simulink model "Charge_1_V1_experiment"  (R2018b)
settings: Solver=FixedStepDiscrete  StartTime=0.0  StopTime=1  FixedStep=0.001  RelTol=1e-3
PreLoadFcn:
  | librarySetup
  | eval([bdroot,'_startup']) %Calling [modelName]_startup.m
undefined symbols (not defined in the file or in its folder): A0, A1, Car1__Authorize, Car2_Authorize, CON2, CON3, CON4, Control_Mode_In, CurrentSP, D10, D12, D13, D2, D3, D4, D5, D6, D7, D8, Free_Charge, Frequency_High_Point, Frequency_Low_Point, Frequency_Mid_high, Frequency_Mid_low, HVol_High_Point, HVol_Low_Point, HVol_Mid_high, HVol_Mid_low, HVoltage_Factor, SeconCar_ThreePhase, V_Current_five, V_Current_four, V_Current_one, V_Current_six, V_Current_three, V_Current_two, V_Frequency, V_MaxPliot, V_MinPliot, Vol_High_Point, Vol_Low_Point, Vol_Mid_high, Vol_Mid_low, Voltage_Factor, Voltage_Mode_Test
libraries: simulink x324, HANcoder_STM32_Target x30, powerlib_meascontrol x8, simulink_extras x2
(part 1 of 13)
CloseFcn:
  | rtwprivate ssgencode ModelCloseRequest mytest
settings Model: Creator=Jason van Kolfschoten  LastModifiedBy=TrungNguyen
settings SolverCC: PositivePriorityOrder=on
settings DataIOCC: LimitDataPoints=on  SaveFormat=Array  SignalLoggingSaveFormat=ModelDataLogs  SaveOutput=off  SaveTime=off
settings OptimizationCC: BlockReduction=off  DefaultParameterBehavior=Inlined  InlineInvariantSignals=on  ExpressionDepthLimit=2147483647  StateBitsets=on  DataBitsets=on  ZeroExternalMemoryAtStartup=off  ZeroInternalMemoryAtStartup=off  InitFltsAndDblsToZero=on  NoFixptDivByZeroProtection=on  EfficientFloat2IntCast=on  LifeSpan=inf
settings DebuggingCC: SaveWithDisabledLinksMsg=none  SaveWithParameterizedLinksMsg=none  CheckSSInitialOutputMsg=off  UnderspecifiedInitializationDetection=Classic  MergeDetectMultiDrivingBlocksExec=none  SignalResolutionControl=TryResolveAll  SolverPrmCheckMsg=warning  InheritedTsInSrcMsg=none  MultiTaskDSMMsg=warning  MultiTaskCondExecSysMsg=none  ParameterPrecisionLossMsg=none  FcnCallInpInsideContextMsg=warning  StateNameClashWarn=warning  SFUnexpectedBacktrackingDiag=warning  SFNoUnconditionalDefaultTransitionDiag=warning  SFExecutionAtInitializationDiag=none
settings HardwareCC: ProdBitPerPointer=32  ProdBitPerSizeT=32  ProdBitPerPtrDiffT=32  ProdLargestAtomicFloat=None  ProdIntDivRoundTo=Undefined  ProdWordSize=32  ProdHWDeviceType=Generic->32-bit Embedded Processor  TargetEndianess=LittleEndian  TargetHWDeviceType=Infineon->TriCore
settings ModelReferenceCC: PropagateSignalLabelsOutOfModel=off
settings SFSimCC: SimUseLocalCustomCode=off  MATLABDynamicMemAlloc=off
settings RTWCC: SystemTargetFile=ert.tlc  MakeCommand=make_rtw SHELL= HANcoder_PORTABLE=1 HANcoder_BOOTLOADER=1  TemplateMakefile=STM32_E407_gcc.tmf  Description=Real-Time Workshop Embedded Coder (no auto configuration)  RTWUseLocalCustomCode=off
settings CodeAppCC: ForceParamTrailComments=on  IgnoreCustomStorageClasses=off  SimulinkDataObjDesc=on  CustomSymbolStrGlobalVar=rt$N$M  CustomSymbolStrType=$N$M  CustomSymbolStrFcn=$N$M$F  CustomSymbolStrMacro=$N$M  InsertBlockDesc=on  StateflowObjectComments=on  InternalIdentifier=Classic
settings ERTTargetCC: TargetFcnLib=ansi_tfl_tmw.mat  MultiwordLength=2048  IncludeMdlTerminateFcn=off  SuppressErrorStatus=on  SupportNonFinite=off  GenerateASAP2=on  InlinedParameterPlacement=NonHierarchical  ERTCustomFileTemplate=example_file_process.tlc  ConvertIfToSwitch=off  SuppressUnreachableDefaultCases=off  IndentSize=4
settings ConfigComp: CovMetricSettings=dw  CovHtmlReporting=on  CovSaveCumulativeToWorkspaceVar=on  CovSaveSingleToWorkspaceVar=on  CovExternalEMLEnable=off  DVMaxProcessTime=600  DVDisplayUnsatisfiableObjectives=on  DVAutomaticStubbing=off  DVModelCoverageObjectives=MCDC  DVMaxTestCaseSteps=500  DVTestSuiteOptimization=CombinedObjectives  DVDetectActiveLogic=on  DVSaveHarnessModel=on

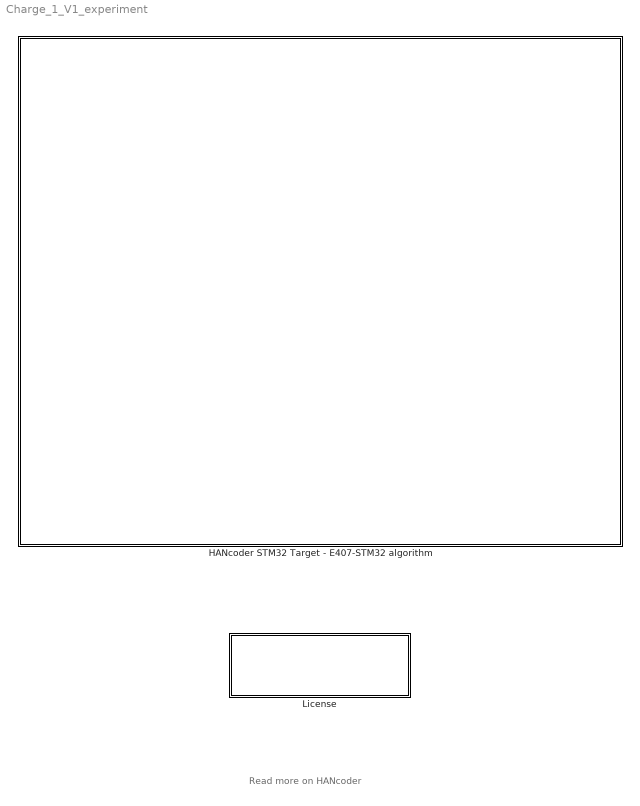
== system Charge_1_V1_experiment ==
  note: Read more on HANcoder
  HANcoder STM32 Target - E407-STM32 algorithm : Subsystem  mask(TopLevelSubsystem){}
      settings: CopyFcn=HANcoderChecks('Copy');  NameChangeFcn=HANcoderChecks('NameChangeE407');  MoveFcn=HANcoderChecks('MoveE407');
      mask Display: image(imread('STM32_E407_HAN.jpg'))
  License : Subsystem  mask(License){}
      settings: NameChangeFcn=HANcoderChecks('NameChangeLicenseBlock');  OpenFcn=winopen('License.pdf')  MoveFcn=HANcoderChecks('MoveLicenseBlock');
      mask Display: disp(['End-User License Agreement\n','please read before use']);

== system Charge_1_V1_experiment/HANcoder STM32 Target - E407-STM32 algorithm ==
  note: Chang current SP for each of charger
  note: Spare_Digital A4(from particle)
  Authorized card : Subsystem
  Car1 : Subsystem
  Car2 : Subsystem
  Config : Subsystem
  Counter Limited1 : simulink/Sources/Counter Limited  uplimit=20  tsamp=0.001
  Current_SP : Subsystem
  Delay : Delay  DelayLength=1  InitialCondition=0
  Delay1 : Delay  DelayLength=1  InitialCondition=0
  Energy Meter : Subsystem
  Partclie_SP_Receive : Subsystem
  Subsystem : Subsystem
  Terminator{,1..12} (13 alike) : Terminator
  wires:
  Current_SP/2(PWM_Out2) -> Car2/3(PWM_Signal)
  Delay1/1 -> Current_SP/18(Charge_state2)
  Car2/1(Out1) -> Delay1/1
  Current_SP/1(PWM_Out1) -> Car1/3(PWM_signal)
  Delay/1 -> Current_SP/17(Charge_state)
  Car1/1(state) -> Delay/1
  Counter Limited1/1 -> Partclie_SP_Receive/1(In1)
  Subsystem/2(V_Auth) -> Terminator2/1
  Subsystem/5(V_Current1) -> Terminator4/1
  Subsystem/6(V_Current2) -> Terminator5/1
  Subsystem/7(V_Current3) -> Terminator6/1
  Subsystem/8(V_Current4) -> Terminator7/1
  Subsystem/9(V_Current5) -> Terminator8/1
  Subsystem/10(V_Current6) -> Terminator9/1
  Subsystem/11(V_MaxPilot) -> Terminator10/1
  Subsystem/12(V_MinPilot) -> Terminator11/1
  Subsystem/4(2ndcarThreephase) -> Terminator3/1
  Authorized card/1(Sysstartcar1) -> Car1/1(System_Start)
  Authorized card/2(Sysstartcar2) -> Car2/1(" System_Start")
  Subsystem/3(V_Auth1) -> Terminator12/1
  Authorized card/3(RFID_Read) -> Car2/2(Read_RFID), Car1/2(RFID)
  Authorized card/4(2_Car_Connected) -> Current_SP/1(2_carConnected)
  Energy Meter/1(Current Phase 1) -> Current_SP/2(Cuurent1)
  Energy Meter/2(Current phase 2) -> Current_SP/3(Current2)
  Energy Meter/3(Current phase 3) -> Current_SP/4(Current3)
  Energy Meter/4(Current phase 4) -> Current_SP/5(Cuurent4)
  Energy Meter/5(Current phase 5) -> Current_SP/6(Current5)
  Energy Meter/6(Current phase 6) -> Current_SP/7(Current6)
  Energy Meter/7(vol1) -> Current_SP/8(vol1)
  Energy Meter/8(vol2) -> Current_SP/9(vol2)
  Energy Meter/9(vol3) -> Current_SP/10(vol3)
  Energy Meter/10(vol4) -> Current_SP/11(vol4)
  Energy Meter/11(vol5) -> Current_SP/12(vol5)
  Energy Meter/12(vol6) -> Current_SP/13(vol6)
  Partclie_SP_Receive/1(Particle_SP1) -> Current_SP/15(ParticleSP)
  Partclie_SP_Receive/2(Particle_SP2) -> Current_SP/16(ParticleSP2)
  Energy Meter/13(Fre) -> Terminator/1
  Subsystem/1(V_Fre) -> Current_SP/14(Frequency), Terminator1/1

== system Charge_1_V1_experiment/License ==

== system Charge_1_V1_experiment/HANcoder STM32 Target - E407-STM32 algorithm/Authorized card ==
  Constant : Constant  Value=Free_Charge  OutDataTypeStr=boolean  SampleTime=-1
  Digital Input : HANcoder_STM32_Target/STM32-E407/Digital Inputs/Digital Input  Tag=HANcoder_TARGET_STM32_E407  pinID=CON2 - A2 - 5V Tolerant  config=Floating  tsamp=0.01
      settings: SourceProductName=HANcoder STM32 Target
  Digital Input1 : HANcoder_STM32_Target/STM32-E407/Digital Inputs/Digital Input  Tag=HANcoder_TARGET_STM32_E407  pinID=CON2 - A3 - 5V Tolerant  config=Floating  tsamp=0.01
      settings: SourceProductName=HANcoder STM32 Target
  Digital Input2 : HANcoder_STM32_Target/STM32-E407/Digital Inputs/Digital Input  Tag=HANcoder_TARGET_STM32_E407  pinID=CON2 - A4 - 5V Tolerant  config=Floating  tsamp=0.001
      settings: SourceProductName=HANcoder STM32 Target
  Logical Operator : Logic  AllPortsSameDT=off  OutDataTypeStr=boolean
  Logical Operator1 : Logic  Operator=OR  AllPortsSameDT=off  OutDataTypeStr=boolean
  Logical Operator2 : Logic  Operator=OR  AllPortsSameDT=off  OutDataTypeStr=boolean
  Sysstartcar1 : Outport
  Sysstartcar2 : Outport  Port=2
  RFID_Read : Outport  Port=3
  2_Car_Connected : Outport  Port=4
  wires:
  Logical Operator2/1 -> Sysstartcar2/1, Logical Operator/1  "Enable_card2"
  Logical Operator1/1 -> Logical Operator/2, Sysstartcar1/1  "Enable_card1"
  Logical Operator/1 -> 2_Car_Connected/1
  Digital Input2/1 -> RFID_Read/1  "RFID_Read"
  Constant/1 -> Logical Operator2/1, Logical Operator1/2
  Digital Input/1 -> Logical Operator1/1
  Digital Input1/1 -> Logical Operator2/2

== system Charge_1_V1_experiment/HANcoder STM32 Target - E407-STM32 algorithm/Car1 ==
  note: Force system start and remove locking actuator
  System_Start : Inport
  RFID : Inport  Port=2
  PWM_signal : Inport  Port=3
  Chart1 : Stateflow chart  TreatAsAtomicUnit=on
  Motorlock controll : Subsystem
  Output leds : Subsystem
  PWM : Subsystem
  Pilotcar1 : Subsystem
  Terminator : Terminator
  Terminator1 : Terminator
  delaytime : Subsystem
  state : Outport
  wires:
  Chart1/2(Pwm) -> PWM/2(Current_SP)
  Pilotcar1/2(Charger_level_min) -> Chart1/2(Minvalue)
  PWM_signal/1 -> Chart1/3(inPWM)
  Pilotcar1/1(Charger_level_max) -> Chart1/1(Maxvalue)
  Chart1/1(Switch) -> Terminator/1, delaytime/1(In1)  "LockCar1On"
  System_Start/1 -> Chart1/4(Start)
  delaytime/1(Lockoutput) -> Terminator1/1  "LockCar1off"
  delaytime/2(Switch_output) -> PWM/1(Switch)  "SwitchCar1"
  Chart1/3(State) -> Output leds/1(State), state/1  "Car1State"
  RFID/1 -> Output leds/2(RFID)

== system Charge_1_V1_experiment/HANcoder STM32 Target - E407-STM32 algorithm/Car2 ==
  " System_Start" : Inport
  Read_RFID : Inport  Port=2
  PWM_Signal : Inport  Port=3
  Chart1 : Stateflow chart  TreatAsAtomicUnit=on
  Motorlock controll : Subsystem
  Output leds : Subsystem
  PWM : Subsystem
  Pilotcar2 : Subsystem
  Terminator : Terminator
  Terminator1 : Terminator
  delaytime : Subsystem
  Out1 : Outport
  wires:
  delaytime/2(Switch_output) -> PWM/1(Switch)  "SwitchCar2"
  delaytime/1(Lockoutput) -> Terminator1/1  "LockCar2off"
  " System_Start"/1 -> Chart1/4(Start)
  Chart1/1(Switch) -> Terminator/1, delaytime/1(In1)  "LockCar2On"
  Pilotcar2/1(Charger_level_max) -> Chart1/1(Maxvalue)  "Maxpilotcar2"
  PWM_Signal/1 -> Chart1/3(inPWM)
  Pilotcar2/2(Charger_level_min) -> Chart1/2(Minvalue)  "Minpilotcar2"
  Chart1/2(Pwm) -> PWM/2(Current_SP)
  Chart1/3(State) -> Out1/1, Output leds/1(State)  "Car2State"
  Read_RFID/1 -> Output leds/2(RFID)

== system Charge_1_V1_experiment/HANcoder STM32 Target - E407-STM32 algorithm/Config ==
  Base Sample Time config : HANcoder_STM32_Target/STM32-E407/System Config/Base Sample Time config  Tag=HANcoder_TARGET_STM32_E407  Description=HANcoder Target STM32-E407 blockset version 0.5  baseSampleTime=1  extraStack=5000
      settings: SourceProductName=HANcoder STM32 Target
  Build settings : HANcoder_STM32_Target/STM32-E407/System Config/Build settings  Tag=HANcoder_TARGET_STM32_E407  AutoASAP2add=on  AutoFlash=Ethernet
      settings: SourceProductName=HANcoder STM32 Target
  Custom ID config : HANcoder_STM32_Target/STM32-E407/System Config/Custom ID config  Tag=HANcoder_TARGET_STM32_E407  softID=softwareID  softNUM=1
      settings: SourceProductName=HANcoder STM32 Target
  Ethernet config : HANcoder_STM32_Target/STM32-E407/System Config/Ethernet config  Tag=HANcoder_TARGET_STM32_E407  ip1=169  ip2=254  ip3=19  ip4=63  nm1=255  nm2=255  nm3=0  nm4=0  gw1=169  gw2=254  gw3=1  gw4=1
      settings: SourceProductName=HANcoder STM32 Target
  System information : Subsystem
  XCP on TCP/IP config : HANcoder_STM32_Target/STM32-E407/System Config/XCP on TCP//IP config  Tag=HANcoder_TARGET_STM32_E407  port=1000
      settings: SourceProductName=HANcoder STM32 Target

== system Charge_1_V1_experiment/HANcoder STM32 Target - E407-STM32 algorithm/Current_SP ==
  note: When 2 car had been connected, current need to reduce to 16A first
  note: Control Mode: 1 : Particle SP
      | 			   2: Frequency
      | 			  3: Hantune_SP
      | 			  4: Free_Charge
      | 			  5: Voltage_Mode
  2_carConnected : Inport
  Cuurent1 : Inport  Port=2
  Current2 : Inport  Port=3
  Current3 : Inport  Port=4
  Cuurent4 : Inport  Port=5
  Current5 : Inport  Port=6
  Current6 : Inport  Port=7
  vol1 : Inport  Port=8
  vol2 : Inport  Port=9
  vol3 : Inport  Port=10
  vol4 : Inport  Port=11
  vol5 : Inport  Port=12
  vol6 : Inport  Port=13
  Frequency : Inport  Port=14
  ParticleSP : Inport  Port=15  OutDataTypeStr=single
  ParticleSP2 : Inport  Port=16  OutDataTypeStr=single
  Charge_state : Inport  Port=17
  Charge_state2 : Inport  Port=18
  Constant1 : Constant  Value=Control_Mode_In  OutDataTypeStr=single  SampleTime=0.01
  Current_Limit1 : Subsystem
  Subsystem1 : Subsystem
  Subsystem2 : Subsystem
  Voltage_input : Subsystem
  Voltage_input1 : Subsystem
  Voltage_testblock : Subsystem
  PWM_Out1 : Outport
  PWM_Out2 : Outport  Port=2
  wires:
  Subsystem1/1(PWM_Out1) -> PWM_Out1/1
  Charge_state/1 -> Subsystem1/9(Sys_charge)
  Charge_state2/1 -> Subsystem2/7(Sys_charge)
  Subsystem2/1(PWM_Out1) -> PWM_Out2/1
  Frequency/1 -> Subsystem2/8(Frequency)
  Constant1/1 -> Subsystem2/10(Control_Mode)  "Mode"
  2_carConnected/1 -> Current_Limit1/1(2_carConnected)
  Current_Limit1/4(Current_Limit) -> Subsystem2/1(Current_Limit)
  Cuurent1/1 -> Current_Limit1/2(In1)
  Current2/1 -> Current_Limit1/3(In2)
  Current3/1 -> Current_Limit1/4(In3)
  Current_Limit1/5(Frequency_Conditionnd) -> Subsystem2/2(Condition)
  ParticleSP2/1 -> Subsystem2/9(Particleinput)
  ParticleSP/1 -> Subsystem1/10(Particleenter1)
  Subsystem2/2(2carConnect_O) -> Subsystem1/4(2ndCarConnected)
  Subsystem2/3(Fre_O) -> Subsystem1/5(Frequency)
  Subsystem2/6(Control_Mode_Out) -> Subsystem1/8(Control_mode)
  Subsystem2/5(Condition_O) -> Subsystem1/7(Fre_Cond)
  Subsystem2/4(Current_Limit_O) -> Subsystem1/6(CurrenLimitCar1)
  Cuurent4/1 -> Current_Limit1/5(In4)
  Current5/1 -> Current_Limit1/6(In5)
  Current6/1 -> Current_Limit1/7(In6)
  Current_Limit1/6(Out4) -> Subsystem2/3(In4)
  Current_Limit1/7(Out5) -> Subsystem2/4(In5)
  Current_Limit1/8(Out6) -> Subsystem2/5(In6)
  Current_Limit1/9(2_carConnected_O) -> Subsystem2/6(2carConnect)
  Current_Limit1/1(Out1) -> Subsystem1/1(Phase1)
  Current_Limit1/2(Out2) -> Subsystem1/2(Phase2)
  Current_Limit1/3(Out3) -> Subsystem1/3(Phase3)
  Subsystem2/7(3phasecar2) -> Current_Limit1/9(3phasecar2)
  Subsystem1/2(3phasecar1) -> Current_Limit1/8(3phasecar1)
  vol2/1 -> Voltage_input/2(In2)
  vol3/1 -> Voltage_input/3(In3)
  vol4/1 -> ?
  vol5/1 -> Voltage_input1/2(In2)
  vol6/1 -> Voltage_input1/3(In3)
  Voltage_input/1(Out1) -> Subsystem1/11(Voltage)  "Voltage_level_check"
  Voltage_input1/1(Out1) -> Subsystem2/11(Voltage_in)  "Voltage_level_check_1"
  Voltage_testblock/1(Vol) -> Voltage_input1/1(In1), Voltage_input/1(In1)

== system Charge_1_V1_experiment/HANcoder STM32 Target - E407-STM32 algorithm/Energy Meter ==
  Counter Limited1 : simulink/Sources/Counter Limited  uplimit=1400  tsamp=0.001
  Energy_Meter : Subsystem
  Energy_Meter_Recieve : Subsystem
  Energymeter_Request : Subsystem
  Particle : Subsystem
  Current Phase 1 : Outport
  Current phase 2 : Outport  Port=2
  Current phase 3 : Outport  Port=3
  Current phase 4 : Outport  Port=4
  Current phase 5 : Outport  Port=5
  Current phase 6 : Outport  Port=6
  vol1 : Outport  Port=7
  vol2 : Outport  Port=8
  vol3 : Outport  Port=9
  vol4 : Outport  Port=10
  vol5 : Outport  Port=11
  vol6 : Outport  Port=12
  Fre : Outport  Port=13
  wires:
  Counter Limited1/1 -> Energy_Meter_Recieve/1(In1)
  Energy_Meter_Recieve/1(Current Phase 1) -> Current Phase 1/1
  Energy_Meter_Recieve/2(Current phase 2) -> Current phase 2/1
  Energy_Meter_Recieve/3(Current phase 3) -> Current phase 3/1
  Energy_Meter_Recieve/4(Current phase 4) -> Current phase 4/1
  Energy_Meter_Recieve/5(Current phase 5) -> Current phase 5/1
  Energy_Meter_Recieve/6(Current phase 6) -> Current phase 6/1
  Energy_Meter_Recieve/13(Frequency) -> Fre/1
  Energy_Meter_Recieve/7(vol1) -> vol1/1
  Energy_Meter_Recieve/8(vol2) -> vol2/1
  Energy_Meter_Recieve/12(vol6) -> vol6/1
  Energy_Meter_Recieve/11(vol5) -> vol5/1
  Energy_Meter_Recieve/10(vol4) -> vol4/1
  Energy_Meter_Recieve/9(vol3) -> vol3/1

== system Charge_1_V1_experiment/HANcoder STM32 Target - E407-STM32 algorithm/Partclie_SP_Receive ==
  In1 : Inport
  SP1 : Subsystem
  Particle_SP1 : Outport  OutDataTypeStr=single  SampleTime=0.1
  Particle_SP2 : Outport  Port=2  OutDataTypeStr=single  SampleTime=0.1
  wires:
  In1/1 -> SP1/1(In1)
  SP1/1(Out1) -> Particle_SP1/1
  SP1/2(Out2) -> Particle_SP2/1

== system Charge_1_V1_experiment/HANcoder STM32 Target - E407-STM32 algorithm/Subsystem ==
  Constant : Constant  Value=V_Frequency  OutDataTypeStr=single  SampleTime=-1
  Constant1 : Constant  Value=SeconCar_ThreePhase  SampleTime=-1
  Constant10 : Constant  Value=V_MinPliot  SampleTime=-1
  Constant11 : Constant  Value=Car2_Authorize  OutDataTypeStr=boolean  SampleTime=0.01
  Constant2 : Constant  Value=V_Current_one  SampleTime=-1
  Constant3 : Constant  Value=V_Current_two  SampleTime=-1
  Constant4 : Constant  Value=V_Current_three  SampleTime=-1
  Constant5 : Constant  Value=V_Current_four  SampleTime=-1
  Constant6 : Constant  Value=V_Current_five  SampleTime=-1
  Constant7 : Constant  Value=V_Current_six  SampleTime=-1
  Constant8 : Constant  Value=Car1__Authorize  OutDataTypeStr=boolean  SampleTime=0.01
  Constant9 : Constant  Value=V_MaxPliot  SampleTime=-1
  Fre_testblock : Subsystem
  Terminator : Terminator
  V_Fre : Outport
  V_Auth : Outport  Port=2
  V_Auth1 : Outport  Port=3
  2ndcarThreephase : Outport  Port=4
  V_Current1 : Outport  Port=5
  V_Current2 : Outport  Port=6
  V_Current3 : Outport  Port=7
  V_Current4 : Outport  Port=8
  V_Current5 : Outport  Port=9
  V_Current6 : Outport  Port=10
  V_MaxPilot : Outport  Port=11
  V_MinPilot : Outport  Port=12
  wires:
  Constant/1 -> Terminator/1
  Constant8/1 -> V_Auth/1
  Constant1/1 -> 2ndcarThreephase/1
  Constant2/1 -> V_Current1/1
  Constant3/1 -> V_Current2/1
  Constant4/1 -> V_Current3/1
  Constant5/1 -> V_Current4/1
  Constant6/1 -> V_Current5/1
  Constant7/1 -> V_Current6/1
  Constant9/1 -> V_MaxPilot/1
  Constant10/1 -> V_MinPilot/1
  Constant11/1 -> V_Auth1/1
  Fre_testblock/1(Fre) -> V_Fre/1

== system Charge_1_V1_experiment/HANcoder STM32 Target - E407-STM32 algorithm/Car1/Motorlock controll ==
  LockOn : Inport
  LockOff : Inport  Port=2
  Digital Output : HANcoder_STM32_Target/STM32-E407/Digital Outputs/Digital Output  Tag=HANcoder_TARGET_STM32_E407  pinID=CON PD - 3  config=Push pull  tsamp=-1
      settings: SourceProductName=HANcoder STM32 Target
  Digital Output1 : HANcoder_STM32_Target/STM32-E407/Digital Outputs/Digital Output  Tag=HANcoder_TARGET_STM32_E407  pinID=CON PD - 4  config=Push pull  tsamp=-1
      settings: SourceProductName=HANcoder STM32 Target
  Edge Detector : powerlib_meascontrol/Logic/Edge Detector  model=Rising  ic=0  Ts=0.4
      settings: SourceProductName=Simscape Electrical  SourceProductBaseCode=PS
  Edge Detector1 : powerlib_meascontrol/Logic/Edge Detector  model=Falling  ic=0  Ts=0.4
      settings: SourceProductName=Simscape Electrical  SourceProductBaseCode=PS
  wires:
  LockOn/1 -> Edge Detector/1
  LockOff/1 -> Edge Detector1/1
  Edge Detector/1 -> Digital Output/1
  Edge Detector1/1 -> Digital Output1/1

== system Charge_1_V1_experiment/HANcoder STM32 Target - E407-STM32 algorithm/Car1/Output leds ==
  State : Inport
  RFID : Inport  Port=2
  Compensated_value : Lookup_n-D  NumberOfTableDimensions=1  BreakpointsForDimension1=[1, 2,3, 4, 5,6,7 ]  Table=[1,0,0,0,0,1,1]  TableDataTypeStr=single  ExtrapMethod=Clip  InternalRulePriority=Speed  RndMeth=Simplest  InputSameDT=on
  Compensated_value1 : Lookup_n-D  NumberOfTableDimensions=1  BreakpointsForDimension1=[1, 2,3, 4, 5,6,7 ]  Table=[1,1,1,0,0,0,1]  TableDataTypeStr=single  ExtrapMethod=Clip  InternalRulePriority=Speed  RndMeth=Simplest  InputSameDT=on
  Compensated_value2 : Lookup_n-D  NumberOfTableDimensions=1  BreakpointsForDimension1=[1, 2,3, 4, 5,6,7 ]  Table=[1,0,1,1,1,0,0]  TableDataTypeStr=single  ExtrapMethod=Clip  InternalRulePriority=Speed  RndMeth=Simplest  InputSameDT=on
  Data Type Conversion : DataTypeConversion  OutDataTypeStr=boolean
  Data Type Conversion1 : DataTypeConversion  OutDataTypeStr=boolean
  Data Type Conversion2 : DataTypeConversion  OutDataTypeStr=boolean
  Digital Output : HANcoder_STM32_Target/STM32-E407/Digital Outputs/Digital Output  Tag=HANcoder_TARGET_STM32_E407  pinID=CON3 - D2  config=Push pull  tsamp=-1
      settings: SourceProductName=HANcoder STM32 Target
  Digital Output1 : HANcoder_STM32_Target/STM32-E407/Digital Outputs/Digital Output  Tag=HANcoder_TARGET_STM32_E407  pinID=CON3 - D3  config=Push pull  tsamp=-1
      settings: SourceProductName=HANcoder STM32 Target
  Digital Output2 : HANcoder_STM32_Target/STM32-E407/Digital Outputs/Digital Output  Tag=HANcoder_TARGET_STM32_E407  pinID=CON3 - D4  config=Push pull  tsamp=-1
      settings: SourceProductName=HANcoder STM32 Target
  Logical Operator : Logic  Operator=OR  AllPortsSameDT=off  OutDataTypeStr=boolean
  Logical Operator1 : Logic  Operator=OR  AllPortsSameDT=off  OutDataTypeStr=boolean
  Logical Operator2 : Logic  Operator=OR  AllPortsSameDT=off  OutDataTypeStr=boolean
  wires:
  State/1 -> Compensated_value/1, Compensated_value2/1, Compensated_value1/1
  ? -> ?  "idle - white state A - blue State B - cyan State C - green State D - green State E - red State F - pink"
  Compensated_value/1 -> Data Type Conversion/1  "State_Test"
  Compensated_value2/1 -> Data Type Conversion2/1  "State_Test_2"
  Compensated_value1/1 -> Data Type Conversion1/1  "State_Test_1"
  Logical Operator/1 -> Digital Output/1
  Data Type Conversion/1 -> Logical Operator/2
  Logical Operator1/1 -> Digital Output2/1
  Logical Operator2/1 -> Digital Output1/1
  Data Type Conversion2/1 -> Logical Operator2/2
  Data Type Conversion1/1 -> Logical Operator1/2
  RFID/1 -> Logical Operator2/1, Logical Operator1/1, Logical Operator/1

== system Charge_1_V1_experiment/HANcoder STM32 Target - E407-STM32 algorithm/Car1/PWM ==
  note: PWM Fre ???
  Switch : Inport
  Current_SP : Inport  Port=2
  Abs : Abs
  Digital Output : HANcoder_STM32_Target/STM32-E407/Digital Outputs/Digital Output  Tag=HANcoder_TARGET_STM32_E407  pinID=CON4 - D8  config=Push pull  tsamp=0.001
      settings: SourceProductName=HANcoder STM32 Target
  Gain3 : Gain  Gain=1023  OutDataTypeStr=uint16
  PWM Duty Cycle : HANcoder_STM32_Target/STM32-E407/PWM Outputs/PWM Duty Cycle  Tag=HANcoder_TARGET_STM32_E407  pinID=CON4 - D12  tsamp=0.001
      settings: SourceProductName=HANcoder STM32 Target
  PWM Init : Subsystem  Tag=HANcoder_TARGET_STM32_E407  AncestorBlock=HANcoder_STM32_Target/STM32-E407/PWM Outputs/PWM Init  mask(Pulse Width Modulation Initialization){moduleID=TIM3:   D12 & D11 & n/a & n/a, frequency=1000, alignment=Edge aligned, enableIRQoutput=off, ch1On=on, ch1Pol=Active high, ch1Inv=off, ch2On=off, ch2Pol=Active high, ch2Inv=off, ch3On=off, ch3Pol=Active high, ch3Inv=off, ch4On=off, ch4Pol=Active high, ch4Inv=off}
      mask prompts: moduleID "PWM module"; frequency "Signal frequency [Hz]"; alignment "Signal alignment"; enableIRQoutput "Enable IRQ output"; ch1On "Generate PWM signal on channel 1"; ch1Pol "Select signal polarity"; ch1Inv "Enable inverted signal on additional output pin"; ch2On "Generate PWM signal on channel 2"; ch2Pol "Select signal polarity"; ch2Inv "Enable inverted signal on additional output pin"; ch3On "Generate PWM signal on channel 3"; ch3Pol "Select signal polarity"; ch3Inv "Enable inverted signal on additional output pin"; ch4On "Generate PWM signal on channel 4"; ch4Pol "Select signal polarity"; ch4Inv "Enable inverted signal on additional output pin"
      mask help:
      | Function
      | ========
      | A 'PWM Init' block configures one of the STM32 timer modules for PWM
      | functionality, allowing a PWM signal to be generated on up to 4 timer
      | channels and their associated output pins.
      |
      | Parameters
      | ==========
      | General - PWM module:
      |   Select the PWM module to use. The name in the combo box contains
      |   information about which pins on the target belong to this timer module.
      |   Also the first pin corresponds with the first channel and so on:
      |   TIMx: Ch1 & Ch2 & Ch3...
      |
      | General - Signal frequency:
      |   Determines the signal frequency in Hz. If you click 'Apply' after entering
      |   the desired frequency it will automatically be adjusted to the closest
      |   supported value.
      |
      | General - Signal Aligment:
      |   Determines the aligment of the signal. It can either be edge aligned or
      |   center aligned.
      |
      | General - Enable IRQ output
      |   Controls whether or not the IRQ output is available.
      |
      | Channel x - Generate PWM signal on channel x:
      |   Enable to configure the channel for PWM functionality so that the PWM signal
      |   is outputted on the channel's associated microcontroller pin.
      |
      | Channel x - Signal polarity:
      |   Selects the polarity of the signal.
      |
      | Channel x - Enable inverted signal on additional output pin:
      |   When enabled, a second PWM signal will be generated on an additional
      |   microcontroller pin where the signal is an exact inversion of the first signal.
      mask init:
      | moduleIDInfoStr = sfcn_pwmout_init_mcb(2, moduleID, frequency, alignment, enableIRQoutput, ch1On, ch2On, ch3On, ch4On, ch1Pol, ch2Pol, ch3Pol, ch4Pol, ch1Inv, ch2Inv, ch3Inv, ch4Inv);
      settings: CopyFcn=sfcn_pwmout_init_chk();  MoveFcn=drawLogos
      mask Help: web('sfcn_pwmout_init.html');
      mask TypeOptions moduleID: TIM1:   PE12 & PE14 & PE16 & PE17 + N-channels PE11 & PE13 & PE15 | TIM2:   D13 & n/a & n/a & n/a | TIM3:   D12 & D11 & n/a & n/a | TIM4:   PD15 & PD16 &n/a & n/a | TIM8:   UEXT3 & UEXT4 & n/a & n/a | TIM9:   D4 & D5 & n/a & n/a | TIM10: A1 & n/a & n/a & n/a | TIM11: A2 & n/a & n/a & n/a | TIM13: A3 & n/a & n/a & n/a | TIM14: A4 & n/a & n/a & n/a
      mask Callback moduleID: sfcn_pwmout_init_chk();
      mask TypeOptions alignment: Edge aligned | Center aligned
      mask TypeOptions ch1Pol: Active high | Active low
      mask TypeOptions ch2Pol: Active high | Active low
      mask TypeOptions ch3Pol: Active high | Active low
      mask TypeOptions ch4Pol: Active high | Active low
      mask Display: fprintf('PWM Init\n%s', moduleIDInfoStr);patch([195 201 201],[8 14 2],[1 0 0]);patch([203 203 209],[14 2 8],[0 0 0.35]);
  wires:
  Gain3/1 -> PWM Duty Cycle/1
  Current_SP/1 -> Abs/1  "Current_Input_car1"
  Abs/1 -> Gain3/1
  Switch/1 -> Digital Output/1

== system Charge_1_V1_experiment/HANcoder STM32 Target - E407-STM32 algorithm/Car1/Pilotcar1 ==
  note: Increase sampling time of Base model
  note: 12V 3.08
      | 9v 2.744
      | 6v 2.404
      | 3v 2.065
      | 0v 1.725
      | -12V 0.366
  1-D Lookup Table1 : Lookup_n-D  NumberOfTableDimensions=1  BreakpointsForDimension1=[-12.5, -10.5]  Table=[-0.2, -1]  TableDataTypeStr=single  ExtrapMethod=Clip  InternalRulePriority=Speed  RndMeth=Simplest  InputSameDT=on
  3.3v 12 bit resolution convert : Gain  Gain=(3.3)/4096  OutDataTypeStr=single
  Add : Sum  Inputs=+-
  Add1 : Sum  Inputs=+-
  Add2 : Sum
  Add3 : Sum
  Analog Input : HANcoder_STM32_Target/STM32-E407/Analog Inputs/Analog Input  Tag=HANcoder_TARGET_STM32_E407  pinID=CON2 - A1  tsamp=-1  filtered=off
      settings: SourceProductName=HANcoder STM32 Target
  Compare To Constant : simulink/Logic and Bit Operations/Compare To Constant  relop===  const=500  OutDataTypeStr=boolean
  Compensated_value : Lookup_n-D  NumberOfTableDimensions=1  BreakpointsForDimension1=[0, 1.5 , 7.5, 10.5, 12.5 ]  Table=[0, 1, 1, 1, 2 ]  TableDataTypeStr=single  ExtrapMethod=Clip  InternalRulePriority=Speed  RndMeth=Simplest  InputSameDT=on
  Constant2 : Constant  Value=1.724953329  OutDataTypeStr=single  SampleTime=-1
  Counter Limited1 : simulink/Sources/Counter Limited  uplimit=1000  tsamp=-1
  Data Type Conversion1 : DataTypeConversion  OutDataTypeStr=single
  Gain : Gain  Gain=8.89967033  OutDataTypeStr=single
  Gain2 : Gain  Gain=8.89967033
  MVA_Filter : Subsystem
  Max : simulink/Math Operations/MinMax Running Resettable  Function=max  vinit=0.0
  Max_filter : Subsystem
  MinMax Running Resettable : simulink/Math Operations/MinMax Running Resettable  Function=min  vinit=12.0
  Min_filter : Subsystem
  Related with resistorValue(Mid point value) Convert back to maximum of 12V resolution : Constant  Value=1.724953329  OutDataTypeStr=single  SampleTime=-1
  Charger_level_max : Outport  SampleTime=0.001
  Charger_level_min : Outport  Port=2  SampleTime=0.001
  wires:
  Analog Input/1 -> Data Type Conversion1/1  "PilotCar1Raw"
  Data Type Conversion1/1 -> 3.3v 12 bit resolution convert/1
  3.3v 12 bit resolution convert/1 -> MinMax Running Resettable/1, Max/1
  Counter Limited1/1 -> Compare To Constant/1
  Related with resistorValue(Mid point value) Convert back to maximum of 12V resolution/1 -> Add/2
  Add/1 -> Gain/1
  Add1/1 -> Gain2/1
  Constant2/1 -> Add1/2
  Max/1 -> MVA_Filter/1(In1)
  MVA_Filter/1(Out1) -> Add/1
  Max_filter/1(Out1) -> Compensated_value/1, Add2/1
  Gain2/1 -> Min_filter/1(In1)
  MinMax Running Resettable/1 -> Add1/1
  Compensated_value/1 -> Add2/2
  Add2/1 -> Charger_level_max/1  "Max_Pilot"
  Min_filter/1(Out1) -> Add3/1, 1-D Lookup Table1/1
  1-D Lookup Table1/1 -> Add3/2
  Compare To Constant/1 -> Max/2, MinMax Running Resettable/2
  Gain/1 -> Max_filter/1(In1)
  Add3/1 -> Charger_level_min/1  "Min_Pilot"

== system Charge_1_V1_experiment/HANcoder STM32 Target - E407-STM32 algorithm/Car1/delaytime ==
  In1 : Inport
  Off Delay : powerlib_meascontrol/Logic/On Delay  DelayType=Off delay  delay=2  ic=1  Ts=2
      settings: SourceProductName=Simscape Electrical
  On Delay : powerlib_meascontrol/Logic/On Delay  DelayType=On delay  delay=2  ic=0  Ts=2
      settings: SourceProductName=Simscape Electrical
  Lockoutput : Outport
  Switch_output : Outport  Port=2
  wires:
  On Delay/1 -> Off Delay/1, Switch_output/1
  Off Delay/1 -> Lockoutput/1
  In1/1 -> On Delay/1

== system Charge_1_V1_experiment/HANcoder STM32 Target - E407-STM32 algorithm/Car2/Motorlock controll ==
  note: Relay on at Zero
  LockOn : Inport
  Lockoff : Inport  Port=2
  Digital Output : HANcoder_STM32_Target/STM32-E407/Digital Outputs/Digital Output  Tag=HANcoder_TARGET_STM32_E407  pinID=CON PD - 10  config=Push pull  tsamp=-1
      settings: SourceProductName=HANcoder STM32 Target
  Digital Output1 : HANcoder_STM32_Target/STM32-E407/Digital Outputs/Digital Output  Tag=HANcoder_TARGET_STM32_E407  pinID=CON PD - 6  config=Push pull  tsamp=-1
      settings: SourceProductName=HANcoder STM32 Target
  Edge Detector : powerlib_meascontrol/Logic/Edge Detector  model=Rising  ic=0  Ts=0.4
      settings: SourceProductName=Simscape Electrical  SourceProductBaseCode=PS
  Edge Detector1 : powerlib_meascontrol/Logic/Edge Detector  model=Falling  ic=0  Ts=0.4
      settings: SourceProductName=Simscape Electrical  SourceProductBaseCode=PS
  wires:
  Lockoff/1 -> Edge Detector1/1
  Edge Detector1/1 -> Digital Output1/1
  LockOn/1 -> Edge Detector/1
  Edge Detector/1 -> Digital Output/1

== system Charge_1_V1_experiment/HANcoder STM32 Target - E407-STM32 algorithm/Car2/Output leds ==
  State : Inport
  RFID : Inport  Port=2
  Compensated_value : Lookup_n-D  NumberOfTableDimensions=1  BreakpointsForDimension1=[1, 2,3, 4, 5,6,7 ]  Table=[1,0,0,0,0,1,1]  TableDataTypeStr=single  ExtrapMethod=Clip  InternalRulePriority=Speed  RndMeth=Simplest  InputSameDT=on
  Compensated_value1 : Lookup_n-D  NumberOfTableDimensions=1  BreakpointsForDimension1=[1, 2,3, 4, 5,6,7 ]  Table=[1,1,1,0,0,0,1]  TableDataTypeStr=single  ExtrapMethod=Clip  InternalRulePriority=Speed  RndMeth=Simplest  InputSameDT=on
  Compensated_value2 : Lookup_n-D  NumberOfTableDimensions=1  BreakpointsForDimension1=[1, 2,3, 4, 5,6,7 ]  Table=[1,0,1,1,1,0,0]  TableDataTypeStr=single  ExtrapMethod=Clip  InternalRulePriority=Speed  RndMeth=Simplest  InputSameDT=on
  Data Type Conversion : DataTypeConversion  OutDataTypeStr=boolean
  Data Type Conversion1 : DataTypeConversion  OutDataTypeStr=boolean
  Data Type Conversion2 : DataTypeConversion  OutDataTypeStr=boolean
  Digital Output : HANcoder_STM32_Target/STM32-E407/Digital Outputs/Digital Output  Tag=HANcoder_TARGET_STM32_E407  pinID=CON3 - D5  config=Push pull  tsamp=-1
      settings: SourceProductName=HANcoder STM32 Target
  Digital Output1 : HANcoder_STM32_Target/STM32-E407/Digital Outputs/Digital Output  Tag=HANcoder_TARGET_STM32_E407  pinID=CON3 - D6  config=Push pull  tsamp=-1
      settings: SourceProductName=HANcoder STM32 Target
  Digital Output2 : HANcoder_STM32_Target/STM32-E407/Digital Outputs/Digital Output  Tag=HANcoder_TARGET_STM32_E407  pinID=CON3 - D7  config=Push pull  tsamp=-1
      settings: SourceProductName=HANcoder STM32 Target
  Logical Operator : Logic  Operator=OR  AllPortsSameDT=off  OutDataTypeStr=boolean
  Logical Operator1 : Logic  Operator=OR  AllPortsSameDT=off  OutDataTypeStr=boolean
  Logical Operator2 : Logic  Operator=OR  AllPortsSameDT=off  OutDataTypeStr=boolean
  wires:
  Data Type Conversion2/1 -> Logical Operator2/2
  Data Type Conversion1/1 -> Logical Operator1/2
  Data Type Conversion/1 -> Logical Operator/2
  Compensated_value1/1 -> Data Type Conversion1/1
  Compensated_value2/1 -> Data Type Conversion2/1
  Compensated_value/1 -> Data Type Conversion/1
  ? -> ?  "idle - white state A - blue State B - cyan State C - green State D - green State E - red State F - pink"
  State/1 -> Compensated_value1/1, Compensated_value2/1, Compensated_value/1
  Logical Operator1/1 -> Digital Output2/1
  Logical Operator/1 -> Digital Output/1
  Logical Operator2/1 -> Digital Output1/1
  RFID/1 -> Logical Operator/1, Logical Operator1/1, Logical Operator2/1

== system Charge_1_V1_experiment/HANcoder STM32 Target - E407-STM32 algorithm/Car2/PWM ==
  note: PWM Fre ???
  Switch : Inport
  Current_SP : Inport  Port=2
  Abs : Abs
  Digital Output : HANcoder_STM32_Target/STM32-E407/Digital Outputs/Digital Output  Tag=HANcoder_TARGET_STM32_E407  pinID=CON4 - D10  config=Push pull  tsamp=0.001
      settings: SourceProductName=HANcoder STM32 Target
  Gain3 : Gain  Gain=1023  OutDataTypeStr=uint16
  PWM Duty Cycle : HANcoder_STM32_Target/STM32-E407/PWM Outputs/PWM Duty Cycle  Tag=HANcoder_TARGET_STM32_E407  pinID=CON4 - D13  tsamp=0.001
      settings: SourceProductName=HANcoder STM32 Target
  PWM Init : Subsystem  Tag=HANcoder_TARGET_STM32_E407  AncestorBlock=HANcoder_STM32_Target/STM32-E407/PWM Outputs/PWM Init  mask(Pulse Width Modulation Initialization){moduleID=TIM2:   D13 & n/a & n/a & n/a, frequency=1000, alignment=Edge aligned, enableIRQoutput=off, ch1On=on, ch1Pol=Active high, ch1Inv=off, ch2On=off, ch2Pol=Active high, ch2Inv=off, ch3On=off, ch3Pol=Active high, ch3Inv=off, ch4On=off, ch4Pol=Active high, ch4Inv=off}
      mask prompts: moduleID "PWM module"; frequency "Signal frequency [Hz]"; alignment "Signal alignment"; enableIRQoutput "Enable IRQ output"; ch1On "Generate PWM signal on channel 1"; ch1Pol "Select signal polarity"; ch1Inv "Enable inverted signal on additional output pin"; ch2On "Generate PWM signal on channel 2"; ch2Pol "Select signal polarity"; ch2Inv "Enable inverted signal on additional output pin"; ch3On "Generate PWM signal on channel 3"; ch3Pol "Select signal polarity"; ch3Inv "Enable inverted signal on additional output pin"; ch4On "Generate PWM signal on channel 4"; ch4Pol "Select signal polarity"; ch4Inv "Enable inverted signal on additional output pin"
      mask help:
      | Function
      | ========
      | A 'PWM Init' block configures one of the STM32 timer modules for PWM
      | functionality, allowing a PWM signal to be generated on up to 4 timer
      | channels and their associated output pins.
      |
      | Parameters
      | ==========
      | General - PWM module:
      |   Select the PWM module to use. The name in the combo box contains
      |   information about which pins on the target belong to this timer module.
      |   Also the first pin corresponds with the first channel and so on:
      |   TIMx: Ch1 & Ch2 & Ch3...
      |
      | General - Signal frequency:
      |   Determines the signal frequency in Hz. If you click 'Apply' after entering
      |   the desired frequency it will automatically be adjusted to the closest
      |   supported value.
      |
      | General - Signal Aligment:
      |   Determines the aligment of the signal. It can either be edge aligned or
      |   center aligned.
      |
      | General - Enable IRQ output
      |   Controls whether or not the IRQ output is available.
      |
      | Channel x - Generate PWM signal on channel x:
      |   Enable to configure the channel for PWM functionality so that the PWM signal
      |   is outputted on the channel's associated microcontroller pin.
      |
      | Channel x - Signal polarity:
      |   Selects the polarity of the signal.
      |
      | Channel x - Enable inverted signal on additional output pin:
      |   When enabled, a second PWM signal will be generated on an additional
      |   microcontroller pin where the signal is an exact inversion of the first signal.
      mask init:
      | moduleIDInfoStr = sfcn_pwmout_init_mcb(2, moduleID, frequency, alignment, enableIRQoutput, ch1On, ch2On, ch3On, ch4On, ch1Pol, ch2Pol, ch3Pol, ch4Pol, ch1Inv, ch2Inv, ch3Inv, ch4Inv);
      settings: CopyFcn=sfcn_pwmout_init_chk();  MoveFcn=drawLogos
      mask Help: web('sfcn_pwmout_init.html');
      mask TypeOptions moduleID: TIM1:   PE12 & PE14 & PE16 & PE17 + N-channels PE11 & PE13 & PE15 | TIM2:   D13 & n/a & n/a & n/a | TIM3:   D12 & D11 & n/a & n/a | TIM4:   PD15 & PD16 &n/a & n/a | TIM8:   UEXT3 & UEXT4 & n/a & n/a | TIM9:   D4 & D5 & n/a & n/a | TIM10: A1 & n/a & n/a & n/a | TIM11: A2 & n/a & n/a & n/a | TIM13: A3 & n/a & n/a & n/a | TIM14: A4 & n/a & n/a & n/a
      mask Callback moduleID: sfcn_pwmout_init_chk();
      mask TypeOptions alignment: Edge aligned | Center aligned
      mask TypeOptions ch1Pol: Active high | Active low
      mask TypeOptions ch2Pol: Active high | Active low
      mask TypeOptions ch3Pol: Active high | Active low
      mask TypeOptions ch4Pol: Active high | Active low
      mask Display: fprintf('PWM Init\n%s', moduleIDInfoStr);patch([195 201 201],[8 14 2],[1 0 0]);patch([203 203 209],[14 2 8],[0 0 0.35]);
  wires:
  Abs/1 -> Gain3/1
  Current_SP/1 -> Abs/1  "Current_input_car2"
  Gain3/1 -> PWM Duty Cycle/1
  Switch/1 -> Digital Output/1

== system Charge_1_V1_experiment/HANcoder STM32 Target - E407-STM32 algorithm/Car2/Pilotcar2 ==
  note: 12V 3.08
      | 9v 2.744
      | 6v 2.404
      | 3v 2.065
      | 0v 1.725
      | -12V 0.366
  note: Increase sampling time of Base model
  1-D Lookup Table1 : Lookup_n-D  NumberOfTableDimensions=1  BreakpointsForDimension1=[-12.5, -10.5]  Table=[-0.2, -1]  TableDataTypeStr=single  ExtrapMethod=Clip  InternalRulePriority=Speed  RndMeth=Simplest  InputSameDT=on
  3.3v 12 bit resolution convert : Gain  Gain=(3.3)/4096  OutDataTypeStr=single
  Add : Sum  Inputs=+-
  Add1 : Sum  Inputs=+-
  Add2 : Sum
  Add3 : Sum
  Analog Input : HANcoder_STM32_Target/STM32-E407/Analog Inputs/Analog Input  Tag=HANcoder_TARGET_STM32_E407  pinID=CON2 - A0  tsamp=-1  filtered=off
      settings: SourceProductName=HANcoder STM32 Target
  Compare To Constant : simulink/Logic and Bit Operations/Compare To Constant  relop===  const=500  OutDataTypeStr=boolean
  Compensated_value : Lookup_n-D  NumberOfTableDimensions=1  BreakpointsForDimension1=[0, 1.5 , 7.5, 10.5, 12.5 ]  Table=[0, 1, 1, 1, 2 ]  TableDataTypeStr=single  ExtrapMethod=Clip  InternalRulePriority=Speed  RndMeth=Simplest  InputSameDT=on
  Constant2 : Constant  Value=1.724953329  OutDataTypeStr=single  SampleTime=-1
  Counter Limited1 : simulink/Sources/Counter Limited  uplimit=1000  tsamp=-1
  Data Type Conversion1 : DataTypeConversion  OutDataTypeStr=single
  Gain : Gain  Gain=8.89967033  OutDataTypeStr=single
  Gain2 : Gain  Gain=8.89967033
  MVA_Filter : Subsystem
  Max : simulink/Math Operations/MinMax Running Resettable  Function=max  vinit=0.0
  Max_filter : Subsystem
  MinMax Running Resettable : simulink/Math Operations/MinMax Running Resettable  Function=min  vinit=12.0
  Min_filter : Subsystem
  Related with resistorValue(Mid point value) Convert back to maximum of 12V resolution : Constant  Value=1.724953329  OutDataTypeStr=single  SampleTime=-1
  Charger_level_max : Outport  SampleTime=0.001
  Charger_level_min : Outport  Port=2  SampleTime=0.001
  wires:
  Add3/1 -> Charger_level_min/1
  Gain/1 -> Max_filter/1(In1)
  Compare To Constant/1 -> MinMax Running Resettable/2, Max/2
  1-D Lookup Table1/1 -> Add3/2
  Min_filter/1(Out1) -> 1-D Lookup Table1/1, Add3/1
  Add2/1 -> Charger_level_max/1
  Compensated_value/1 -> Add2/2
  MinMax Running Resettable/1 -> Add1/1
  Gain2/1 -> Min_filter/1(In1)
  Max_filter/1(Out1) -> Add2/1, Compensated_value/1
  MVA_Filter/1(Out1) -> Add/1
  Max/1 -> MVA_Filter/1(In1)  "Max_out"
  Constant2/1 -> Add1/2
  Add1/1 -> Gain2/1
  Add/1 -> Gain/1
  Related with resistorValue(Mid point value) Convert back to maximum of 12V resolution/1 -> Add/2
  Counter Limited1/1 -> Compare To Constant/1
  3.3v 12 bit resolution convert/1 -> Max/1, MinMax Running Resettable/1
  Data Type Conversion1/1 -> 3.3v 12 bit resolution convert/1
  Analog Input/1 -> Data Type Conversion1/1  "PilotCar2Raw"

== system Charge_1_V1_experiment/HANcoder STM32 Target - E407-STM32 algorithm/Car2/delaytime ==
  In1 : Inport
  Off Delay : powerlib_meascontrol/Logic/On Delay  DelayType=Off delay  delay=2  ic=1  Ts=2
      settings: SourceProductName=Simscape Electrical
  On Delay : powerlib_meascontrol/Logic/On Delay  DelayType=On delay  delay=2  ic=0  Ts=2
      settings: SourceProductName=Simscape Electrical
  Lockoutput : Outport
  Switch_output : Outport  Port=2
  wires:
  In1/1 -> On Delay/1
  Off Delay/1 -> Lockoutput/1
  On Delay/1 -> Off Delay/1, Switch_output/1

== system Charge_1_V1_experiment/HANcoder STM32 Target - E407-STM32 algorithm/Config/System information ==
  note: These blocks check the free memory: stack and heap and the CPU load,
      | this way you can see whether your software demands too much of the microcontroller
  Get CPU load : HANcoder_STM32_Target/STM32-E407/System Management/Get CPU load  Tag=HANcoder_TARGET_STM32_E407  mode=Current CPU load  tsamp=-1
      settings: SourceProductName=HANcoder STM32 Target
  Get free Heap : HANcoder_STM32_Target/STM32-E407/System Management/Get free Heap  Tag=HANcoder_TARGET_STM32_E407  tsamp=-1
      settings: SourceProductName=HANcoder STM32 Target
  Get free Stack : HANcoder_STM32_Target/STM32-E407/System Management/Get free Stack  Tag=HANcoder_TARGET_STM32_E407  taskIdx=Application Control Task  tsamp=-1
      settings: SourceProductName=HANcoder STM32 Target
  Terminator : Terminator
  Terminator1 : Terminator
  Terminator2 : Terminator
  wires:
  Get CPU load/1 -> Terminator1/1  "SI_CPUload"
  Get free Stack/1 -> Terminator/1  "SI_FreeStack"
  Get free Heap/1 -> Terminator2/1  "SI_FreeHeap"

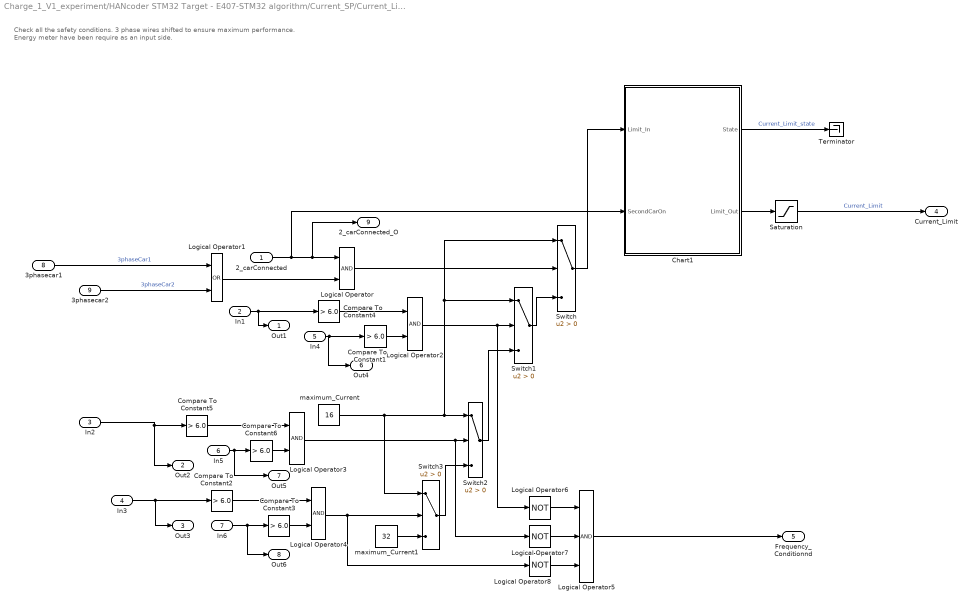
== system Charge_1_V1_experiment/HANcoder STM32 Target - E407-STM32 algorithm/Current_SP/Current_Limit1 ==
  note: Check all the safety conditions. 3 phase wires shifted to ensure maximum performance.
      | Energy meter have been require as an input side.
  2_carConnected : Inport
  In1 : Inport  Port=2
  In2 : Inport  Port=3
  In3 : Inport  Port=4
  In4 : Inport  Port=5
  In5 : Inport  Port=6
  In6 : Inport  Port=7
  3phasecar1 : Inport  Port=8
  3phasecar2 : Inport  Port=9
  Chart1 : Stateflow chart  TreatAsAtomicUnit=on
  Compare To Constant{1..6} (6 alike) : simulink/Logic and Bit Operations/Compare To Constant  relop=>  const=6.0  OutDataTypeStr=boolean
  Logical Operator{,2..4} (4 alike) : Logic  AllPortsSameDT=off  OutDataTypeStr=boolean
  Logical Operator1 : Logic  Operator=OR  AllPortsSameDT=off  OutDataTypeStr=boolean
  Logical Operator5 : Logic  Inputs=3  AllPortsSameDT=off  OutDataTypeStr=boolean
  Logical Operator6 : Logic  Operator=NOT  AllPortsSameDT=off  OutDataTypeStr=boolean
  Logical Operator7 : Logic  Operator=NOT  AllPortsSameDT=off  OutDataTypeStr=boolean
  Logical Operator8 : Logic  Operator=NOT  AllPortsSameDT=off  OutDataTypeStr=boolean
  Saturation : Saturate  UpperLimit=32  LowerLimit=0
  Switch{,1..3} (4 alike) : Switch  Criteria=u2 > Threshold
  Terminator : Terminator
  maximum_Current : Constant  Value=16  SampleTime=-1
  maximum_Current1 : Constant  Value=32  SampleTime=-1
  Out1 : Outport
  Out2 : Outport  Port=2
  Out3 : Outport  Port=3
  Current_Limit : Outport  Port=4
  Frequency_Conditionnd : Outport  Port=5
  Out4 : Outport  Port=6
  Out5 : Outport  Port=7
  Out6 : Outport  Port=8
  2_carConnected_O : Outport  Port=9
  wires:
  Switch2/1 -> Switch1/3
  Logical Operator/1 -> Switch/2
  Logical Operator2/1 -> Logical Operator6/1, Switch1/2
  Logical Operator1/1 -> Logical Operator/2
  3phasecar1/1 -> Logical Operator1/1  "3phaseCar1"
  3phasecar2/1 -> Logical Operator1/2  "3phaseCar2"
  Logical Operator3/1 -> Logical Operator7/1, Switch2/2
  Switch1/1 -> Switch/3
  Logical Operator4/1 -> Switch3/2, Logical Operator8/1
  maximum_Current1/1 -> Switch3/3
  Switch3/1 -> Switch2/3
  In1/1 -> Out1/1, Compare To Constant4/1
  In2/1 -> Out2/1, Compare To Constant5/1
  In3/1 -> Out3/1, Compare To Constant2/1
  Saturation/1 -> Current_Limit/1  "Current_Limit"
  Switch/1 -> Chart1/1(Limit_In)
  Chart1/2(Limit_Out) -> Saturation/1
  Chart1/1(State) -> Terminator/1  "Current_Limit_state"
  2_carConnected/1 -> Chart1/2(SecondCarOn), 2_carConnected_O/1, Logical Operator/1
  maximum_Current/1 -> Switch3/1, Switch/1, Switch1/1, Switch2/1
  Logical Operator8/1 -> Logical Operator5/3
  Logical Operator7/1 -> Logical Operator5/2
  Logical Operator6/1 -> Logical Operator5/1
  Logical Operator5/1 -> Frequency_Conditionnd/1
  Compare To Constant4/1 -> Logical Operator2/1
  Compare To Constant5/1 -> Logical Operator3/1
  Compare To Constant6/1 -> Logical Operator3/2
  Compare To Constant3/1 -> Logical Operator4/2
  Compare To Constant2/1 -> Logical Operator4/1
  Compare To Constant1/1 -> Logical Operator2/2
  In5/1 -> Out5/1, Compare To Constant6/1
  In6/1 -> Out6/1, Compare To Constant3/1
  In4/1 -> Out4/1, Compare To Constant1/1

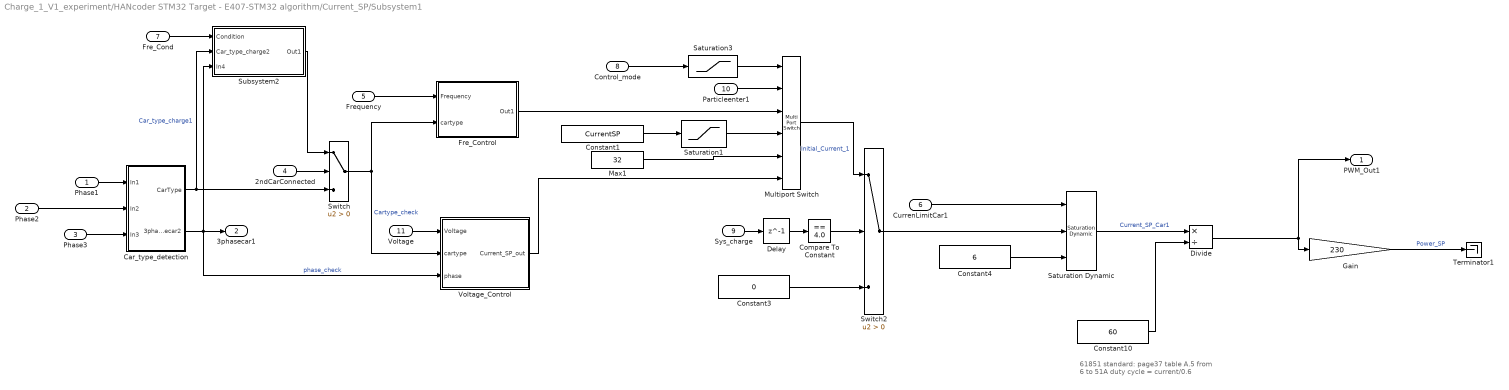
== system Charge_1_V1_experiment/HANcoder STM32 Target - E407-STM32 algorithm/Current_SP/Subsystem1 ==
  note: 61851 standard: page37 table A.5
      | from 6 to 51A duty cycle = current/0.6
  Phase1 : Inport
  Phase2 : Inport  Port=2
  Phase3 : Inport  Port=3
  2ndCarConnected : Inport  Port=4
  Frequency : Inport  Port=5
  CurrenLimitCar1 : Inport  Port=6  OutDataTypeStr=single
  Fre_Cond : Inport  Port=7
  Control_mode : Inport  Port=8
  Sys_charge : Inport  Port=9
  Particleenter1 : Inport  Port=10
  Voltage : Inport  Port=11
  Car_type_detection : Subsystem
  Compare To Constant : simulink/Logic and Bit Operations/Compare To Constant  relop===  const=4.0  OutDataTypeStr=boolean
  Constant1 : Constant  Value=CurrentSP  OutDataTypeStr=single  SampleTime=-1
  Constant10 : Constant  Value=60  OutDataTypeStr=single  SampleTime=-1
  Constant3 : Constant  Value=0  OutDataTypeStr=single  SampleTime=-1
  Constant4 : Constant  Value=6  OutDataTypeStr=single  SampleTime=-1
  Delay : Delay  DelayLength=1  InitialCondition=0
  Divide : Product  Inputs=*/
  Fre_Control : Subsystem
  Gain : Gain  Gain=230  OutDataTypeStr=single
  Max1 : Constant  Value=32  OutDataTypeStr=single  SampleTime=-1
  Multiport Switch : MultiPortSwitch  Inputs=5
  Saturation Dynamic : simulink/Discontinuities/Saturation Dynamic  OutMin=[]  OutMax=[]  OutDataTypeStr=Inherit: Same as second input  OutDataType=fixdt(1, 16)  OutScaling=2^-10  DoSatur=off
  Saturation1 : Saturate  UpperLimit=32  LowerLimit=6
  Saturation3 : Saturate  UpperLimit=5  LowerLimit=1
  Subsystem2 : Subsystem
  Switch : Switch  Criteria=u2 > Threshold
  Switch2 : Switch  Criteria=u2 > Threshold
  Terminator1 : Terminator
  Voltage_Control : Subsystem
  PWM_Out1 : Outport  SampleTime=0.1
  3phasecar1 : Outport  Port=2
  wires:
  Saturation1/1 -> Multiport Switch/4
  Divide/1 -> PWM_Out1/1, Gain/1
  Gain/1 -> Terminator1/1  "Power_SP"
  Car_type_detection/1(CarType) -> Subsystem2/2(Car_type_charge2), Switch/3  "Car_type_charge1"
  Constant1/1 -> Saturation1/1
  Phase1/1 -> Car_type_detection/1(In1)
  Phase3/1 -> Car_type_detection/3(In3)
  Multiport Switch/1 -> Switch2/1  "Initial_Current_1"
  Phase2/1 -> Car_type_detection/2(In2)
  Constant10/1 -> Divide/2
  Sys_charge/1 -> Delay/1
  Delay/1 -> Compare To Constant/1
  Constant3/1 -> Switch2/3
  Compare To Constant/1 -> Switch2/2
  Switch2/1 -> Saturation Dynamic/2
  Saturation Dynamic/1 -> Divide/1  "Current_SP_Car1"
  Constant4/1 -> Saturation Dynamic/3
  CurrenLimitCar1/1 -> Saturation Dynamic/1
  Control_mode/1 -> Saturation3/1
  Particleenter1/1 -> Multiport Switch/2
  Saturation3/1 -> Multiport Switch/1
  Max1/1 -> Multiport Switch/5
  Car_type_detection/2(3phasecar2) -> Voltage_Control/3(phase), Subsystem2/3(In4), 3phasecar1/1  "phase_check"
  Subsystem2/1(Out1) -> Switch/1
  Fre_Cond/1 -> Subsystem2/1(Condition)
  2ndCarConnected/1 -> Switch/2
  Frequency/1 -> Fre_Control/1(Frequency)
  Switch/1 -> Voltage_Control/2(cartype), Fre_Control/2(cartype)  "Cartype_check"
  Fre_Control/1(Out1) -> Multiport Switch/3
  Voltage/1 -> Voltage_Control/1(Voltage)
  Voltage_Control/1(Current_SP_out) -> Multiport Switch/6
